simulink model "sistemaDesacopladoEquivalenteControlPIDposicion"  (R2017a)
settings: Solver=ode45  StartTime=0.0  StopTime=10.0  RelTol=1e-3  EnableMultiTasking=on
values from neighbouring files (symbols this model uses):
  J_m = Jm+(Jl/r^2)    (= 5.65099476805e-06)    [InicializaYconstantes.m]
  Kd = J_m*n*wpos    (= 0.0113019895361)    [InicializaYconstantes.m]
  Ki = J_m*wpos^3    (= 2893.30932124)    [InicializaYconstantes.m]
  Kp = J_m*n*wpos^2    (= 9.04159162887)    [InicializaYconstantes.m]
  r = 314.3008    [InicializaYconstantes.m]
  T_l = Tl/r    (= 0.00499521477515)    [InicializaYconstantes.m]
settings Model: Creator=usuario  LastModifiedBy=usuario
settings DataIOCC: LimitDataPoints=on  SaveFormat=Array
settings OptimizationCC: ExpressionDepthLimit=2147483647  LifeSpan=inf
settings DebuggingCC: UnderspecifiedInitializationDetection=Classic  MergeDetectMultiDrivingBlocksExec=none  SolverPrmCheckMsg=warning  StateNameClashWarn=warning  SFUnexpectedBacktrackingDiag=warning  SFNoUnconditionalDefaultTransitionDiag=warning  SFExecutionAtInitializationDiag=none
settings HardwareCC: ProdBitPerPointer=32  ProdBitPerSizeT=32  ProdBitPerPtrDiffT=32  ProdLargestAtomicFloat=None  ProdIntDivRoundTo=Undefined  ProdEndianess=Unspecified  ProdWordSize=32  ProdHWDeviceType=32-bit Generic
settings ModelReferenceCC: PropagateSignalLabelsOutOfModel=off
settings GRTTargetCC: TargetLangStandard=C89/C90 (ANSI)  GeneratePreprocessorConditionals=Disable all
settings ConfigComp: CovMetricSettings=dw  CovHtmlReporting=on  CovSaveCumulativeToWorkspaceVar=on  CovSaveSingleToWorkspaceVar=on  CovExternalEMLEnable=off

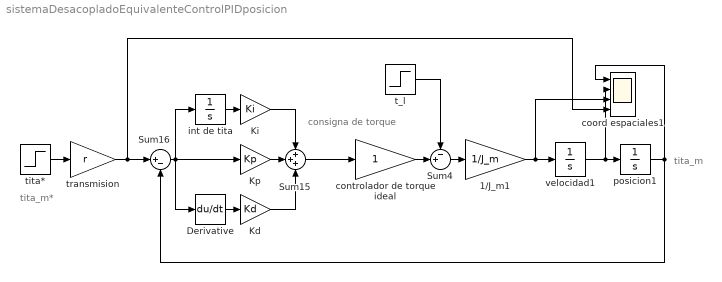
== system sistemaDesacopladoEquivalenteControlPIDposicion ==
  note: tita_m*
  note: tita_m
  note: consigna
      | de torque
  " transmision" : Gain  Gain=r
  1/J_m1 : Gain  Gain=1/J_m
  Derivative : Derivative
  Kd : Gain  Gain=Kd
  Ki : Gain  Gain=Ki
  Kp : Gain  Gain=Kp
  Sum15 : Sum  Inputs=+++
  Sum16 : Sum  Inputs=|+-
  Sum4 : Sum  Inputs=-+|
  "controlador de torque ideal " : Gain
  coord espaciales1 : Scope  NumInputPorts=4
  int de tita : Integrator
  posicion1 : Integrator
  t_l : Step  Time=.3  After=T_l  SampleTime=0
  tita* : Step  Time=0.1  After=2*pi  SampleTime=0
  velocidad1 : Integrator  ContinuousStateAttributes='velocidad'
  wires:
  Ki/1 -> Sum15/1
  Kp/1 -> Sum15/2
  Kd/1 -> Sum15/3
  int de tita/1 -> Ki/1
  Derivative/1 -> Kd/1
  Sum16/1 -> Derivative/1, int de tita/1, Kp/1
  tita*/1 -> " transmision"/1
  " transmision"/1 -> coord espaciales1/4, Sum16/1
  Sum4/1 -> 1/J_m1/1
  t_l/1 -> Sum4/1
  1/J_m1/1 -> velocidad1/1, coord espaciales1/3
  velocidad1/1 -> coord espaciales1/2, posicion1/1
  Sum15/1 -> "controlador de torque ideal "/1
  "controlador de torque ideal "/1 -> Sum4/2
  posicion1/1 -> coord espaciales1/1, Sum16/2
